simulink model "Gekoppelt_Plot"  (R2019b)
settings: Solver=VariableStepAuto  StartTime=0.0  StopTime=100  RelTol=1e-3
undefined symbols (not defined in the file): A1, A2, A3, k1, k2, k3, Kv
libraries: simulink x1
settings Model: OrderedModelArguments=off  Creator=Ogulcan  LastModifiedBy=Ogulcan
settings DebuggingCC: ArithmeticOperatorsInVariantConditions=warning
settings SFSimCC: CustomCodeUndefinedFunction=UseInterfaceOnly

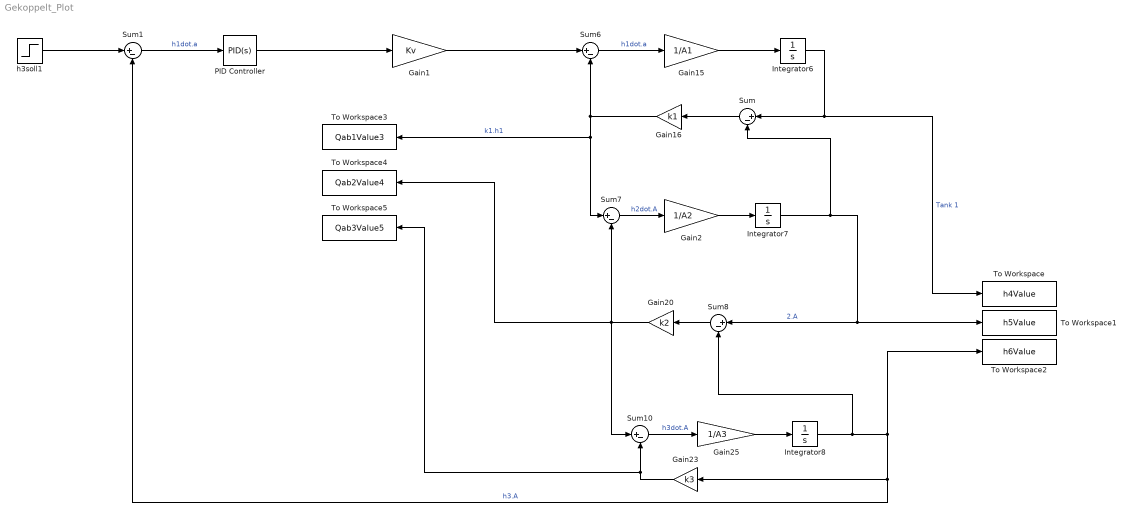
== system Gekoppelt_Plot ==
  Gain1 : Gain  Gain=Kv
  Gain15 : Gain  Gain=1/A1
  Gain16 : Gain  Gain=k1
  Gain2 : Gain  Gain=1/A2
  Gain20 : Gain  Gain=k2
  Gain23 : Gain  Gain=k3
  Gain25 : Gain  Gain=1/A3
  Integrator6 : Integrator
  Integrator7 : Integrator
  Integrator8 : Integrator
  PID Controller : simulink/Continuous/PID Controller  Controller=PID  Form=Ideal  TimeDomain=Continuous-time  SampleTime=-1  IntegratorMethod=Forward Euler  FilterMethod=Forward Euler  ControllerParametersSource=internal  P=2  I=0.05  D=0  UseFilter=on  N=100  TunerSelectOption=Transfer Function Based (PID Tuner App)  InitialConditionSource=internal  InitialConditionForIntegrator=0  InitialConditionForFilter=0  DifferentiatorICPrevScaledInput=0  ExternalReset=none  TrackingMode=off  Kt=1  LimitOutput=off  UpperSaturationLimit=inf  LowerSaturationLimit=-inf  LinearizeAsGain=on  AntiWindupMode=none  Kb=1  POutMin=[]  POutMax=[]  IOutMin=[]  IOutMax=[]  DOutMin=[]  DOutMax=[]  NOutMin=[]  NOutMax=[]  SumOutMin=[]  SumOutMax=[]  SaturationOutMin=[]  SaturationOutMax=[]  PParamMin=[]  PParamMax=[]  IParamMin=[]  IParamMax=[]  DParamMin=[]  DParamMax=[]  NParamMin=[]  NParamMax=[]  KbParamMin=[]  KbParamMax=[]  KtParamMin=[]  KtParamMax=[]  KbOutMin=[]  KbOutMax=[]  KtOutMin=[]  KtOutMax=[]  IntegratorOutMin=[]  IntegratorOutMax=[]  FilterOutMin=[]  FilterOutMax=[]  SumI1OutMin=[]  SumI1OutMax=[]  SumI2OutMin=[]  SumI2OutMax=[]  SumI3OutMin=[]  SumI3OutMax=[]  SumI4OutMin=[]  SumI4OutMax=[]  SumDOutMin=[]  SumDOutMax=[]  DifferentiatorOutMin=[]  DifferentiatorOutMax=[]  FilterDiffOutCoefMin=[]  FilterDiffOutCoefMax=[]  ReciprocalOutMin=[]  ReciprocalOutMax=[]  SumDenOutMin=[]  SumDenOutMax=[]  SumNumOutMin=[]  SumNumOutMax=[]  DivideOutMin=[]  DivideOutMax=[]  IntegratorContinuousStateAttributes=''  IntegratorStateMustResolveToSignalObject=off  IntegratorRTWStateStorageClass=Auto  FilterContinuousStateAttributes=''  FilterStateMustResolveToSignalObject=off  FilterRTWStateStorageClass=Auto  ParallelPVariant=Passthrough  IdealPVariant=InternalParameters  IVariant=InternalParameters  DVariant=InternalParameters  IntegratorVariant=Continuous  SatVariant=Disabled  AWVariant=Passthrough  PCopyVariant=Disabled  TRVariant=Disabled  FdbkBlocksVariant=Forward  IdealPFdbkVariant=Disabled  SatFdbkVariant=Disabled  DerivativeFilterVariant=ContFilter  NVariant=InternalParameters  NCopyVariant=Disabled  FilterICVariant=InternalICsFilter  IntegratorICVariant=InternalICs  ExternalResetVariant=Disabled  TRSumVariant=Passthrough  SumFdbkVariant=Disabled  SumVariant=Sum_PID
  Sum{,1,6..8,10} (6 alike) : Sum  Inputs=|+-
  To Workspace : ToWorkspace  VariableName=h4Value  SaveFormat=Timeseries  SampleTime=-1
  To Workspace1 : ToWorkspace  VariableName=h5Value  SaveFormat=Timeseries  SampleTime=-1
  To Workspace2 : ToWorkspace  VariableName=h6Value  SaveFormat=Timeseries  SampleTime=-1
  To Workspace3 : ToWorkspace  VariableName=Qab1Value3  SaveFormat=Timeseries  SampleTime=-1
  To Workspace4 : ToWorkspace  VariableName=Qab2Value4  SaveFormat=Timeseries  SampleTime=-1
  To Workspace5 : ToWorkspace  VariableName=Qab3Value5  SaveFormat=Timeseries  SampleTime=-1
  h3soll1 : Step  After=1000  SampleTime=0
  wires:
  Gain16/1 -> Sum7/1, To Workspace3/1, Sum6/2  "k1.h1"
  Integrator7/1 -> To Workspace1/1, Sum8/1, Sum/2  "2.A"
  Sum6/1 -> Gain15/1  "h1dot.a"
  Gain15/1 -> Integrator6/1
  Integrator6/1 -> To Workspace/1, Sum/1  "Tank 1"
  Gain25/1 -> Integrator8/1
  Sum10/1 -> Gain25/1  "h3dot.A"
  Integrator8/1 -> To Workspace2/1, Sum1/2, Gain23/1, Sum8/2  "h3.A"
  Sum7/1 -> Gain2/1  "h2dot.A"
  Gain2/1 -> Integrator7/1
  Sum/1 -> Gain16/1
  Sum8/1 -> Gain20/1
  Gain20/1 -> To Workspace4/1, Sum7/2, Sum10/1
  Gain1/1 -> Sum6/1
  h3soll1/1 -> Sum1/1
  PID Controller/1 -> Gain1/1
  Sum1/1 -> PID Controller/1  "h1dot.a"
  Gain23/1 -> To Workspace5/1, Sum10/2
